simulink model "Citation"  (Simulink 10.0)
settings: Solver=ode5  StartTime=0.0  StopTime=700  FixedStep=0.01  RelTol=1e-3  EnableMultiTasking=on
values from neighbouring files (symbols this model uses):
  x0 = []    [cessnac550_3d_sfnc.m]
undefined symbols (not defined in the file or in its folder): chord, cv1, cv2, cv3, cv4, deltagmax1, deltagmax2, deltagmax3, deltagmax4, Deng, ealphag, ealphas, g0, hDME, hGS, kt1, kt2, kt3, lh, massinit, matbuaf, matdaf, matdam, matdbbf, matdeaf, matdgaf, matdqaf, matduaf, matdwaw, matedhr, mateif, matelhr, matemhr, matemv1, matemv2, matemve, matetam, mateuaf, matfaaf, matfaxl, matff, matibaf, matibmh, matipaf, matipmh, matiraf, matiuaf, matiwaf, matlaf, matlam, matleaf, matleam, matlgaf, matlqaf, matluaf, matmaaf, matmaam, matmaf, matmam, matmbbf ... (+77)
undefined symbols (not defined in the file): matibb
libraries: simulink x8, vrlib x1
(part 1 of 5)
settings Model: Creator=laurensvaneykeren  LastModifiedBy=mauro  ExtModeTrigMode=oneshot  ExtModeArmWhenConnect=off
settings DataIOCC: SignalLoggingName=sigsOut
settings OptimizationCC: BooleanDataType=off  ExpressionDepthLimit=2147483647
settings DebuggingCC: SaveWithParameterizedLinksMsg=none  SignalResolutionControl=TryResolveAllWithWarning  MultiTaskDSMMsg=warning  MultiTaskCondExecSysMsg=none  FcnCallInpInsideContextMsg=warning  StateNameClashWarn=warning
settings HardwareCC: TargetUnknown=on
settings RTWCC: SystemTargetFile=grt_malloc.tlc  GenCodeOnly=on  TemplateMakefile=grt_malloc_default_tmf
settings GRTTargetCC: UseMalloc=on

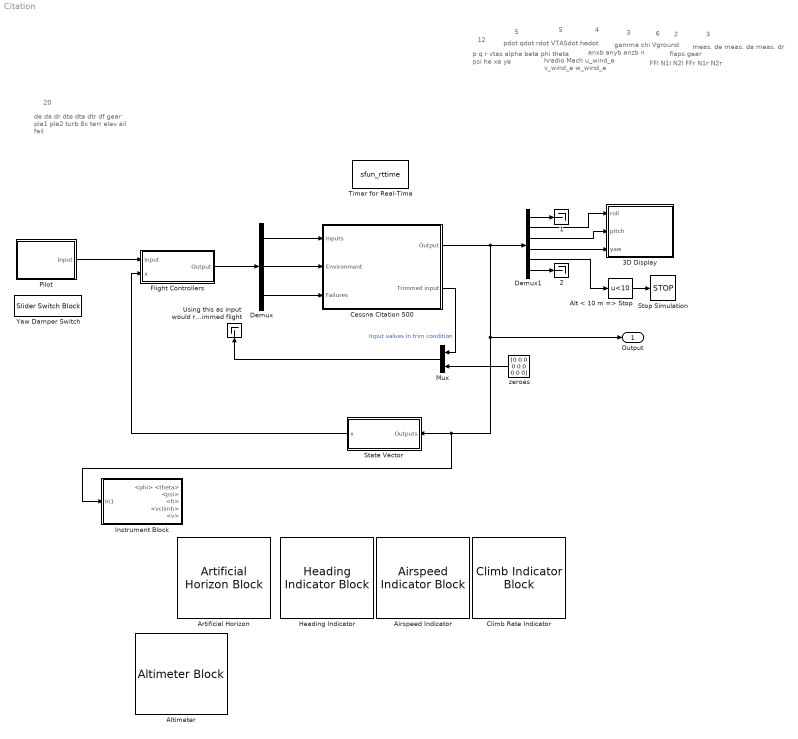
== system Citation ==
  note: de
      | da
      | dr
      | dte
      | dta
      | dtr
      | df
      | gear
      | pla1
      | pla2
      | turb 8x
      | terr elev
      | ail fail
  note: p
      | q
      | r
      | vtas
      | alpha
      | beta
      | phi
      | theta
      | psi
      | he
      | xe
      | ye
  note: pdot
      | qdot
      | rdot
      | VTASdot
      | hedot
  note: hradio
      | Mach
      | u_wind_e
      | v_wind_e
      | w_wind_e
  note: anxb
      | anyb
      | anzb
      | n
  note: gamma
      | chi
      | Vground
  note: flaps
      | gear
  note: FFl
      | N1l
      | N2l
      | FFr
      | N1r
      | N2r
  note: 12
  note: 5
  note: 5
  note: 4
  note: 3
  note: 6
  note: 2
  note: 20
  note: meas. de
      | meas. da
      | meas. dr
  note: 3
  1 : Terminator
  2 : Terminator
  3D Display : Subsystem
  Airspeed Indicator : AirspeedIndicatorBlock  ScaleMax=250  ScaleColors=DataTag1
  Alt < 10 m => Stop : Fcn  Expr=u<10
  Altimeter : AltimeterBlock
  Artificial Horizon : ArtificialHorizonBlock
  Cessna Citation 500 : Subsystem  mask(Citation Aircraft Model){trimdatafile=example.tri}
      mask prompts: trimdatafile "Trim Condition"
      mask init:
      | initcit;
      mask Display:
      | image(imread('Citation.jpg'))
      | port_label('input', 1, 'Inputs')
      | port_label('input', 2, 'Environment')
      | port_label('output', 1, 'Outputs')
      | port_label('output', 2, 'Trim inputs')
  Climb Rate Indicator : ClimbIndicatorBlock  ScaleMax=100
  Demux : Demux  Outputs=[10 9 1]
  Demux1 : Demux  Outputs=[6 1 1 1 1 30]
  Flight Controllers : Subsystem
  Heading Indicator : HeadingIndicatorBlock
  Instrument Block : Subsystem
  Mux : Mux  Inputs=2
  Pilot : Subsystem
  State Vector : Subsystem
  Stop Simulation : Stop
  Timer for Real-Time : S-Function  FunctionName=sfun_rttime  Parameters=1  SFunctionDeploymentMode=off  EnableBusSupport=off
  Using this as input would result in  trimmed flight : Terminator
  Yaw Damper Switch : SliderSwitchBlock  Values=DataTag7
  zeroes : Constant  Value=[0 0 0 0 0 0 0 0 0]
  Output : Outport
  wires:
  zeroes/1 -> Mux/2
  Mux/1 -> Using this as input would result in  trimmed flight/1
  Demux1/1 -> 1/1
  Demux1/2 -> 3D Display/1(roll)
  Demux1/3 -> 3D Display/2(pitch)
  Demux1/4 -> 3D Display/3(yaw)
  Alt < 10 m => Stop/1 -> Stop Simulation/1
  Demux1/6 -> 2/1
  Demux/1 -> Cessna Citation 500/1(Inputs)
  Demux/2 -> Cessna Citation 500/2(Environment)
  Cessna Citation 500/2(Trimmed input) -> Mux/1  "Input values in trim condition"
  Cessna Citation 500/1(Output) -> Demux1/1, Instrument Block/1(In1), State Vector/1(Outputs), Output/1
  Demux/3 -> Cessna Citation 500/3(Failures)
  State Vector/1(x) -> Flight Controllers/2(x)
  Pilot/1(Input) -> Flight Controllers/1(Input)
  Flight Controllers/1(Output) -> Demux/1
  Demux1/5 -> Alt < 10 m => Stop/1

== system Citation/3D Display ==
  roll : Inport
  pitch : Inport  Port=2
  yaw : Inport  Port=3
  Mux1 : Mux
  Position : Subsystem
  S-Function : S-Function  FunctionName=cessnac550_3d_sfnc  SFunctionDeploymentMode=off  EnableBusSupport=off
  Terminator : Terminator
  wires:
  roll/1 -> Mux1/1
  Position/1(Out1) -> Mux1/4
  pitch/1 -> Mux1/2
  yaw/1 -> Mux1/3
  Mux1/1 -> S-Function/1
  S-Function/1 -> Terminator/1

== system Citation/Cessna Citation 500 ==
  note: p
      | q
      | r
      | vtas
      | alpha
      | beta
      | phi
      | theta
      | psi
      | he
      | xe
      | ye
  note: de
      | da
      | dr
      | dte
      | dta
      | dtr
      | df
      | gear
      | pla1
      | pla2
  note: pdot
      | qdot
      | rdot
      | VTASdot
      | hedot
  note: hradio
      | Mach
      | u_wind_e
      | v_wind_e
      | w_wind_e
  note: anxb
      | anyb
      | anzb
      | n
  note: gamma
      | chi
      | Vground
  note: turb 8x
      | terr_elev
  note: flaps
      | gear
  note: de
      | da
      | dr
      | dte
      | dta
      | dtr
      | df
      | gear
      | pla1
      | pla2
  note: FFl
      | N1l
      | N2l
      | FFr
      | N1r
      | N2r
  note: ail fail
  note: meas. de
      | meas. da
      | meas. dr
  Inputs : Inport
  Environment : Inport  Port=2
  Failures : Inport  Port=3
  Actuators : Subsystem
  Citation model DASMAT : Subsystem
  Controllers : Subsystem
  Demux4 : Demux  Outputs=[8 2]
  Mux1 : Mux  Inputs=8
  Mux2 : Mux  Inputs=2
  Selector : Selector  InputPortWidth=12  IndexOptions=Index vector (dialog)  Indices=[10 11 12]  OutputSizes=1
  To File1 : ToFile  Filename=datapross\\data\\defl.mat  MatrixName=defl
  To File2 : ToFile  Filename=datapross\\data\\position.mat  MatrixName=pos
  trim conditions : Subsystem
  ua sel : Selector  IndexOptions=Index vector (dialog)  Indices=[5 6]  OutputSizes=1
  xdot sel : Selector  IndexOptions=Index vector (dialog)  Indices=[1 2 3 4 10]  OutputSizes=1
  yacc sel : Selector  IndexOptions=Index vector (dialog)  Indices=[4 5 6 15]  OutputSizes=1
  yair sel : Selector  IndexOptions=Index vector (dialog)  Indices=[6 9 22 23 24]  OutputSizes=1
  yfp sel : Selector  IndexOptions=Index vector (dialog)  Indices=[1 2 15]  OutputSizes=1
  ypp sel : Selector  IndexOptions=Index vector (dialog)  Indices=[2 3 4 13 14 15]  OutputSizes=1
  Output : Outport
  Trimmed input : Outport  Port=2
  wires:
  Mux1/1 -> Output/1
  Demux4/1 -> Citation model DASMAT/1(ua), ua sel/1
  Demux4/2 -> Citation model DASMAT/2(ut)
  Environment/1 -> Citation model DASMAT/3(Environment)
  Citation model DASMAT/3(yair) -> yair sel/1
  yair sel/1 -> Mux1/3
  Citation model DASMAT/2(xdot) -> xdot sel/1
  yacc sel/1 -> Mux1/4
  Citation model DASMAT/4(yacc) -> yacc sel/1
  yfp sel/1 -> Mux1/5
  Citation model DASMAT/5(yfp) -> yfp sel/1
  Actuators/1(Outputs) -> To File1/1, Demux4/1
  trim conditions/1(ua) -> Mux2/1
  trim conditions/2(ut) -> Mux2/2
  Mux2/1 -> Trimmed input/1
  Controllers/1(control inputs) -> Actuators/1(Inputs)
  ua sel/1 -> Mux1/7
  Citation model DASMAT/6(ypp) -> ypp sel/1
  ypp sel/1 -> Mux1/6
  Inputs/1 -> Controllers/2(inputs)
  Failures/1 -> Actuators/2(Failures)
  Actuators/2(Meas. Defl) -> Mux1/8
  xdot sel/1 -> Mux1/2
  Citation model DASMAT/1(x) -> Selector/1, Mux1/1, Controllers/1(state)
  Selector/1 -> To File2/1

== system Citation/Flight Controllers ==
  Input : Inport
  x : Inport  Port=2
  ANDI : Subsystem
  Classical : Subsystem
  Controller Switch : Subsystem
  INDI : Subsystem
  Multiport Switch : MultiPortSwitch  DataPortForDefault=Additional data port  DiagnosticForDefault=Warning
  To File : ToFile  Filename=datapross\\data\\output.mat  MatrixName=output
  To File1 : ToFile  Filename=datapross\\data\\input.mat  MatrixName=input
  Output : Outport
  wires:
  ANDI/1(Output) -> Multiport Switch/2
  x/1 -> INDI/2(x), Classical/2(x), ANDI/2(x)
  Controller Switch/1(Output) -> Multiport Switch/1
  Input/1 -> To File1/1, ANDI/1(Input), Classical/1(Input), INDI/1(Input), Multiport Switch/5
  INDI/1(Output) -> Multiport Switch/3
  Classical/1(Output) -> Multiport Switch/4
  Multiport Switch/1 -> To File/1, Output/1

== system Citation/Instrument Block ==
  In1 : Inport
  Demux : Demux  Outputs=[3 1 2 1 1 1 1 16 1 13]
  Demux5 : Demux  Outputs=2
  Gain : Gain  Gain=180/pi
  Gain2 : Gain  Gain=180/pi
  MATLAB Function : MATLAB Function  TreatAsAtomicUnit=on
  Mux3 : Mux  Inputs=2
  Mux4 : Mux  Inputs=2
  Product : Product
  Trigonometric Function : Trigonometry
  <phi> <theta> : Outport  VectorParamsAs1DForOutWhenUnconnected=off
  <psi> : Outport  Port=2  VectorParamsAs1DForOutWhenUnconnected=off
  <h> : Outport  Port=3  VectorParamsAs1DForOutWhenUnconnected=off
  <vclimb> : Outport  Port=4  VectorParamsAs1DForOutWhenUnconnected=off
  <v> : Outport  Port=5  VectorParamsAs1DForOutWhenUnconnected=off
  wires:
  Product/1 -> <vclimb>/1
  Mux3/1 -> Gain/1
  Trigonometric Function/1 -> Product/2
  Gain/1 -> Demux5/1
  Demux5/2 -> MATLAB Function/2(theta)
  MATLAB Function/2(theta_r) -> Mux4/2
  Demux5/1 -> MATLAB Function/1(phi)
  MATLAB Function/1(phi_r) -> Mux4/1
  Gain2/1 -> <psi>/1
  In1/1 -> Demux/1
  Mux4/1 -> <phi> <theta>/1
  Demux/2 -> <v>/1, Product/1
  Demux/4 -> Mux3/1
  Demux/5 -> Mux3/2
  Demux/6 -> Gain2/1
  Demux/7 -> <h>/1
  Demux/9 -> Trigonometric Function/1

== system Citation/Pilot ==
  note: de
      | da
      | dr
      | dte
      | dta
      | dtr
      | df
      | gear
      | pla1
      | pla2
      | turb 8x
      | terr elev
      | ail fail
  Joystick : Subsystem
  Mux : Mux  Inputs=13
  da trim : Constant  Value=0
  de trim : Constant  Value=0
  delta flaps : Constant  Value=0
  dr trim : Constant  Value=0
  gear (ON=1/OFF=0) : Constant  Value=0
  terr elev : Constant  Value=0
  turb 8x : Constant  Value=zeros(1,8)
  Input : Outport
  wires:
  Mux/1 -> Input/1
  Joystick/1(delta elevator) -> Mux/1
  Joystick/3(delta rudder) -> Mux/3
  da trim/1 -> Mux/5
  de trim/1 -> Mux/4
  Joystick/2(delta aileron) -> Mux/2
  turb 8x/1 -> Mux/11
  terr elev/1 -> Mux/12
  Joystick/4(Throttle setting) -> Mux/10, Mux/9
  gear (ON=1/OFF=0)/1 -> Mux/8
  dr trim/1 -> Mux/6
  delta flaps/1 -> Mux/7
  Joystick/5(Aileron failure) -> Mux/13

== system Citation/State Vector ==
  note: p
      | q
      | r
      | pdot
      | qdot
      | rdot
      | vtas
      | alpha
      | beta
      | u
      | v
      | w
      | phi
      | theta
      | rho
      | axb
      | ayb
      | azb
      | meas. de
      | meas. da
      | meas. dr
  note: 21
  note: p
      | q
      | r
  note: vtas
      | alpha
      | beta
  note: phi
      | theta
  note: he
  note: anxb
      | anyb
      | anzb
  note: meas. de
      | meas. da
      | meas. dr
  note: p
      | q
      | r
  note: vtas
      | alpha
      | beta
  note: phi
      | theta
  note: pdot
      | qdot
      | rdot
  note: u
      | v
      | w
  note: rho
  note: axb
      | ayb
      | azb
  note: meas. de
      | meas. da
      | meas. dr
  note: 6
  note: pdot
      | qdot
      | rdot
      | VTASdot
      | hedot
  note: 12
  note: meas. de
      | meas. da
      | meas. dr
  note: anxb
      | anyb
      | anzb
      | n
  note: FFl
      | N1l
      | N2l
      | FFr
      | N1r
      | N2r
  note: 5
  note: 3
  note: hradio
      | Mach
      | u_wind_e
      | v_wind_e
      | w_wind_e
  note: 3
  note: flaps
      | gear
  note: p
      | q
      | r
      | vtas
      | alpha
      | beta
      | phi
      | theta
      | psi
      | he
      | xe
      | ye
  note: 5
  note: gamma
      | chi
      | Vground
  note: 2
  note: 4
  Outputs : Inport
  Demux : Demux  Outputs=[3 3 2 1 1 12 3 12 3]
  Demux1 : Demux  Outputs=3
  Derivative : Derivative
  Gain : Gain  Gain=9.807
  MATLAB Function1 : MATLAB Function  TreatAsAtomicUnit=on
  MATLAB Function2 : MATLAB Function  TreatAsAtomicUnit=on
  Mux : Mux  Inputs=8
  Mux1 : Mux  Inputs=3
  Terminator1 : Terminator
  Terminator2 : Terminator
  Terminator3 : Terminator
  x : Outport
  wires:
  Demux/4 -> Terminator1/1
  Outputs/1 -> Demux/1
  Derivative/1 -> Mux/2
  Demux/6 -> Terminator2/1
  Demux/1 -> Mux/1, Derivative/1
  Demux/2 -> Demux1/1, Mux/3
  Demux1/1 -> MATLAB Function1/1(V)
  Demux1/2 -> MATLAB Function1/2(alpha)
  Demux1/3 -> MATLAB Function1/3(beta)
  MATLAB Function1/1(u) -> Mux1/1
  MATLAB Function1/2(v) -> Mux1/2
  MATLAB Function1/3(w) -> Mux1/3
  Mux1/1 -> Mux/4
  Demux/3 -> Mux/5
  MATLAB Function2/1(rho) -> Mux/6
  Demux/5 -> MATLAB Function2/1(h)
  Demux/7 -> Gain/1
  Gain/1 -> Mux/7
  Demux/8 -> Terminator3/1
  Demux/9 -> Mux/8
  Mux/1 -> x/1

== system Citation/3D Display/Position ==
  Mux2 : Mux  Inputs=3
  x : Constant  Value=0
  y : Constant  Value=0
  z : Constant  Value=0
  Out1 : Outport
  wires:
  y/1 -> Mux2/2
  z/1 -> Mux2/3
  x/1 -> Mux2/1
  Mux2/1 -> Out1/1

== system Citation/Cessna Citation 500/Actuators ==
  note: de
      | da
      | dr
      | dte
      | dta
      | dtr
      | df
      | gear
      | pla1
      | pla2
  note: de
      | da
      | dr
      | dte
      | dta
      | dtr
      | df
      | gear
      | pla1
      | pla2
  note: ail fail
  note: meas. de
      | meas. da
      | meas. dr
  Inputs : Inport
  Failures : Inport  Port=2
  Aileron Failure Dynamics : Subsystem
  Demux : Demux  Outputs=10
  Mux : Mux  Inputs=10
  Mux1 : Mux  Inputs=3
  Switch : Switch  Criteria=u2 > Threshold
  da : Subsystem
  da limits : Saturate  UpperLimit=0.65  LowerLimit=-0.65
  de : Subsystem
  de limits : Saturate  UpperLimit=0.26  LowerLimit=-0.35
  dr : Subsystem
  dr limits : Saturate  UpperLimit=0.38  LowerLimit=-0.38
  flaps : Subsystem
  gear : Subsystem
  Outputs : Outport
  Meas. Defl : Outport  Port=2
  wires:
  Inputs/1 -> Demux/1
  Mux/1 -> Outputs/1
  Demux/1 -> de/1(In)
  de/1(Out) -> de limits/1
  da/1(Out) -> da limits/1
  dr/1(Out) -> dr limits/1
  dr limits/1 -> Mux/3, Mux1/3
  de limits/1 -> Mux1/1, Mux/1
  Demux/8 -> gear/1(In)
  Demux/7 -> flaps/1(In)
  Demux/9 -> Mux/9
  Demux/10 -> Mux/10
  flaps/1(Out) -> Mux/7
  gear/1(Out) -> Mux/8
  Demux/4 -> Mux/4
  Demux/5 -> Mux/5
  Demux/6 -> Mux/6
  Failures/1 -> Switch/2
  Demux/3 -> dr/1(In)
  Switch/1 -> Mux/2
  Aileron Failure Dynamics/1(Out) -> Switch/1
  Demux/2 -> da/1(In)
  da limits/1 -> Mux1/2, Switch/3, Aileron Failure Dynamics/1(In)
  Mux1/1 -> Meas. Defl/1

== system Citation/Cessna Citation 500/Citation model DASMAT ==
  ua : Inport
  ut : Inport  Port=2
  Environment : Inport  Port=3
  AIRCRAFT MODEL : Subsystem
  Mux1 : Mux  Inputs=[8 2 8 12 8]
  Terminator_{16..19} (4 alike) : Terminator
  massinit : Constant  Value=massinit
  x : Outport
  xdot : Outport  Port=2
  yair : Outport  Port=3
  yacc : Outport  Port=4
  yfp : Outport  Port=5
  ypp : Outport  Port=6
  wires:
  AIRCRAFT MODEL/13(FMt) -> Terminator_19/1
  Mux1/1 -> yair/1
  AIRCRAFT MODEL/12(FMag) -> Terminator_17/1
  AIRCRAFT MODEL/11(FMa) -> Terminator_18/1
  AIRCRAFT MODEL/7(gust) -> Mux1/5
  AIRCRAFT MODEL/6(wind) -> Mux1/4
  AIRCRAFT MODEL/5(yad2) -> Mux1/3
  AIRCRAFT MODEL/4(yad1) -> Mux1/2
  AIRCRAFT MODEL/3(yatm) -> Mux1/1
  AIRCRAFT MODEL/2(xdot) -> xdot/1
  AIRCRAFT MODEL/1(x) -> x/1
  AIRCRAFT MODEL/10(ys) -> Terminator_16/1
  AIRCRAFT MODEL/9(yfp) -> yfp/1
  AIRCRAFT MODEL/8(yacc) -> yacc/1
  massinit/1 -> AIRCRAFT MODEL/3(massinit)
  ut/1 -> AIRCRAFT MODEL/2(ut)
  ua/1 -> AIRCRAFT MODEL/1(ua)
  Environment/1 -> AIRCRAFT MODEL/4(Environment)
  AIRCRAFT MODEL/14(ypp) -> ypp/1

== system Citation/Cessna Citation 500/Controllers ==
  state : Inport
  inputs : Inport  Port=2
  A/T disabled : Gain  Gain=0  SaturateOnIntegerOverflow=on  OutDataTypeStr=Inherit: Same as input  ParamDataTypeStr=Inherit: Same as input
  Yaw damper : Subsystem
  add controller outputs to pilot inputs : Sum  Inputs=|+|+|+|  SaturateOnIntegerOverflow=on
  auto throttle : Subsystem
  control inputs : Outport
  wires:
  state/1 -> Yaw damper/1(state), auto throttle/1(state)
  inputs/1 -> Yaw damper/2(inputs), add controller outputs to pilot inputs/3, auto throttle/2(inputs)
  add controller outputs to pilot inputs/1 -> control inputs/1
  Yaw damper/1(controller output) -> add controller outputs to pilot inputs/1
  auto throttle/1(controller output) -> A/T disabled/1
  A/T disabled/1 -> add controller outputs to pilot inputs/2

== system Citation/Cessna Citation 500/trim conditions ==
  PLA1/Tx1 : Constant  Value=ut0(1)
  PLA2/Tx2 : Constant  Value=ut0(2)
  control inputs : Mux  Inputs=8
      settings: DisplayOption=signals
  deltaa : Constant  Value=u0(2)
  deltae : Constant  Value=u0(1)
  deltaf : Constant  Value=u0(7)
  deltar : Constant  Value=u0(3)
  deltata : Constant  Value=u0(5)
  deltate : Constant  Value=u0(4)
  deltatr : Constant  Value=u0(6)
  engine inputs : Mux  Inputs=2
      settings: DisplayOption=signals
  lgsw : Constant  Value=u0(8)
  ua : Outport
  ut : Outport  Port=2
  wires:
  deltaf/1 -> control inputs/7  "df"
  engine inputs/1 -> ut/1
  deltatr/1 -> control inputs/6  "dtr"
  deltata/1 -> control inputs/5  "dta"
  control inputs/1 -> ua/1
  PLA1/Tx1/1 -> engine inputs/1  "pla1"
  PLA2/Tx2/1 -> engine inputs/2  "pla2"
  deltae/1 -> control inputs/1  "de"
  deltaa/1 -> control inputs/2  "da"
  deltar/1 -> control inputs/3  "dr"
  deltate/1 -> control inputs/4  "dte"
  lgsw/1 -> control inputs/8  "lg"

== system Citation/Flight Controllers/ANDI ==
  Input : Inport
  x : Inport  Port=2
  ANDI : Subsystem
  Demux : Demux  Outputs=[1 1 1 17]
  Memory : Memory  InitialCondition=[0, 0, 0, 0, 0, 0, 90.0, 0.0560, 0, 89.8590, 0, 5.0352, 0, 0.0037, 1.0065, 0.036, 0, -9.8008, -0.0248, 0, 0]
  Mux2 : Mux  Inputs=2
  Selector1 : Selector  InputPortWidth=3  IndexOptions=Index vector (dialog)  Indices=[2 1 3]  OutputSizes=1
  Output : Outport
  wires:
  Input/1 -> Demux/1
  Selector1/1 -> Mux2/1
  Demux/2 -> ANDI/2(p_ref)
  Demux/4 -> Mux2/2
  Demux/3 -> ANDI/4(beta_ref)
  Demux/1 -> ANDI/3(q_ref)
  Mux2/1 -> Output/1
  Memory/1 -> ANDI/1(x)
  x/1 -> Memory/1
  ANDI/1(Output) -> Selector1/1

== system Citation/Flight Controllers/Classical ==
  Input : Inport
  x : Inport  Port=2
  Classical : Subsystem
  Demux : Demux  Outputs=[1 1 1 17]
  Memory : Memory  InitialCondition=[0, 0, 0, 0, 0, 0, 90.0, 0.0560, 0, 89.8590, 0, 5.0352, 0, 0.0037, 1.0065, 0.036, 0, -9.8008, -0.0248, 0, 0]
  Mux2 : Mux  Inputs=2
  Selector1 : Selector  InputPortWidth=3  IndexOptions=Index vector (dialog)  Indices=[2 1 3]  OutputSizes=1
  Output : Outport
  wires:
  Input/1 -> Demux/1
  Selector1/1 -> Mux2/1
  Demux/2 -> Classical/2(p_ref)
  Demux/4 -> Mux2/2
  Demux/3 -> Classical/4(beta_ref)
  Demux/1 -> Classical/3(q_ref)
  Mux2/1 -> Output/1
  Memory/1 -> Classical/1(x)
  x/1 -> Memory/1
  Classical/1(Output) -> Selector1/1

== system Citation/Flight Controllers/Controller Switch ==
  Gain : Gain  Gain=[1;2;3;4]
  MATLAB Function : MATLAB Function  TreatAsAtomicUnit=on
  Memory : Memory  InitialCondition=1
  Output : Outport
  wires:
  [CSwitch] -> Gain/1
  Gain/1 -> MATLAB Function/1(input)
  MATLAB Function/1(output) -> Memory/1, Output/1
  Memory/1 -> MATLAB Function/2(prev)

== system Citation/Flight Controllers/INDI ==
  Input : Inport
  x : Inport  Port=2
  Demux : Demux  Outputs=[1 1 1 17]
  INDI : Subsystem
  Memory : Memory  InitialCondition=[0, 0, 0, 0, 0, 0, 90.0, 0.0560, 0, 89.8590, 0, 5.0352, 0, 0.0037, 1.0065, 0.036, 0, -9.8008, -0.0248, 0, 0]
  Mux2 : Mux  Inputs=2
  Selector1 : Selector  InputPortWidth=3  IndexOptions=Index vector (dialog)  Indices=[2 1 3]  OutputSizes=1
  Output : Outport
  wires:
  Input/1 -> Demux/1
  Selector1/1 -> Mux2/1
  Demux/2 -> INDI/2(p_ref)
  Demux/4 -> Mux2/2
  Demux/1 -> INDI/3(q_ref)
  Mux2/1 -> Output/1
  Memory/1 -> INDI/1(x)
  x/1 -> Memory/1
  INDI/1(Output) -> Selector1/1
  Demux/3 -> INDI/4(beta_ref)

== system Citation/Pilot/Joystick ==
  note: Button 3
  note: Button 2
  note: raw inputs
      | aileron [-0.6328,0.014,0.72] right+
      | elevator [-0.6973,-0.033,0.5725] backwards+
      | throttle [-0.6407,0,0.5317]bacwards+
      | rudder [-0.56,0.127,0.73] right+
  note: normalize inputs
      | aileron [-1,0,1] left+
      | elevator [-1,0,1] forward+
      | rudder [-1,0,1] left+
      | throttle [-1,0,1] forward+
  note: apply real limits
      | [deg]
      | [%]
  note: Convert to radians
      | [rad]
      | [%]
  Constant : Constant  Value=0
  Constant1 : Constant  Value=0
  Constant2 : Constant
  Constant3 : Constant  Value=0
  Dead Zone : DeadZone  LowerValue=-0.02  UpperValue=0.02  SaturateOnIntegerOverflow=on
  Dead Zone1 : DeadZone  LowerValue=-0.02  UpperValue=0.02  SaturateOnIntegerOverflow=on
  Dead Zone2 : DeadZone  LowerValue=-0.01  UpperValue=0.01  SaturateOnIntegerOverflow=on
  Demux : Demux  Outputs=2
  Demux1 : Demux
  Gain : Gain  Gain=-1  SaturateOnIntegerOverflow=on  OutDataTypeStr=Inherit: Same as input  ParamDataTypeStr=Inherit: Same as input
  Gain1 : Gain  Gain=-1  SaturateOnIntegerOverflow=on  OutDataTypeStr=Inherit: Same as input  ParamDataTypeStr=Inherit: Same as input
  Gain11 : Gain  Gain=pi/180  SaturateOnIntegerOverflow=on  OutDataTypeStr=Inherit: Same as input  ParamDataTypeStr=Inherit: Same as input
  Gain2 : Gain  Gain=-0.5  SaturateOnIntegerOverflow=on  OutDataTypeStr=Inherit: Same as input  ParamDataTypeStr=Inherit: Same as input
  Gain3 : Gain  Gain=-1  SaturateOnIntegerOverflow=on  OutDataTypeStr=Inherit: Same as input  ParamDataTypeStr=Inherit: Same as input
  Gain4 : Gain  Gain=37.24  SaturateOnIntegerOverflow=on  OutDataTypeStr=Inherit: Same as input  ParamDataTypeStr=Inherit: Same as input
  Gain5 : Gain  Gain=20  SaturateOnIntegerOverflow=on  OutDataTypeStr=Inherit: Same as input  ParamDataTypeStr=Inherit: Same as input
  Gain6 : Gain  SaturateOnIntegerOverflow=on  OutDataTypeStr=Inherit: Same as input  ParamDataTypeStr=Inherit: Same as input
  Gain7 : Gain  Gain=22  SaturateOnIntegerOverflow=on  OutDataTypeStr=Inherit: Same as input  ParamDataTypeStr=Inherit: Same as input
  Gain8 : Gain  Gain=pi/180  SaturateOnIntegerOverflow=on  OutDataTypeStr=Inherit: Same as input  ParamDataTypeStr=Inherit: Same as input
  Gain9 : Gain  Gain=pi/180  SaturateOnIntegerOverflow=on  OutDataTypeStr=Inherit: Same as input  ParamDataTypeStr=Inherit: Same as input
  Joystick Input : vrlib/Joystick Input  joyid=1  adjustports=on  forcefeed=off
      settings: SourceProductName=Simulink
  Selector : Selector  InputPortWidth=12  IndexOptions=Index vector (dialog)  Indices=[2 3]  OutputSizes=1
  Selector1 : Selector  InputPortWidth=12  IndexOptions=Index vector (dialog)  Indices=[7 9 11 12]  OutputSizes=1
  Sum{,1..3} (4 alike) : Sum  Inputs=-+|  SaturateOnIntegerOverflow=on
  Switch : Subsystem
  Terminator4 : Terminator
  delta elevator : Outport
  delta aileron : Outport  Port=2
  delta rudder : Outport  Port=3
  Throttle setting : Outport  Port=4
  Aileron failure : Outport  Port=5
  tag scope: CSwitch=global, FSwitch=global
  wires:
  Joystick Input/1 -> Demux1/1
  Joystick Input/2 -> Selector/1, Selector1/1
  Joystick Input/3 -> Terminator4/1
  Demux1/1 -> Sum/2
  Constant/1 -> Sum/1
  Constant1/1 -> Sum1/1
  Demux1/2 -> Sum1/2
  Constant2/1 -> Sum2/1
  Constant3/1 -> Sum3/1
  Sum/1 -> Dead Zone/1
  Gain/1 -> Gain4/1
  Sum1/1 -> Dead Zone1/1
  Gain1/1 -> Gain5/1
  Sum2/1 -> Gain2/1
  Sum3/1 -> Dead Zone2/1
  Gain3/1 -> Gain7/1
  Gain4/1 -> Gain8/1
  Gain5/1 -> Gain9/1
  Gain6/1 -> Throttle setting/1
  Gain7/1 -> Gain11/1
  Gain8/1 -> delta aileron/1
  Gain9/1 -> delta elevator/1
  Gain11/1 -> delta rudder/1
  Gain2/1 -> Gain6/1
  Demux1/4 -> Sum2/2
  Demux1/3 -> Sum3/2
  Dead Zone/1 -> Gain/1
  Dead Zone1/1 -> Gain1/1
  Dead Zone2/1 -> Gain3/1
  Demux/1 -> Switch/1(On)
  Demux/2 -> Switch/2(Off)
  Switch/1(Switch out) -> [FSwitch], Aileron failure/1
  Selector/1 -> Demux/1
  Selector1/1 -> [CSwitch]

== system Citation/Cessna Citation 500/Actuators/Aileron Failure Dynamics ==
  In : Inport
  Constant : Constant  Value=0.28
  Gain : Gain  Gain=0.5
  Sum : Sum  Inputs=|++
  Out : Outport
  wires:
  In/1 -> Gain/1
  Constant/1 -> Sum/2
  Gain/1 -> Sum/1
  Sum/1 -> Out/1

== system Citation/Cessna Citation 500/Actuators/da ==
  In : Inport
  Gain : Gain  Gain=13  SaturateOnIntegerOverflow=on  OutDataTypeStr=Inherit: Same as input  ParamDataTypeStr=Inherit: Same as input
  Integrator : Integrator  InitialCondition=u0(2)
  Sum : Sum  Inputs=|+-  SaturateOnIntegerOverflow=on
  Out : Outport
  wires:
  Integrator/1 -> Out/1, Sum/2
  In/1 -> Sum/1
  Sum/1 -> Gain/1
  Gain/1 -> Integrator/1

== system Citation/Cessna Citation 500/Actuators/de ==
  In : Inport
  Gain : Gain  Gain=13  SaturateOnIntegerOverflow=on  OutDataTypeStr=Inherit: Same as input  ParamDataTypeStr=Inherit: Same as input
  Integrator : Integrator  InitialCondition=u0(1)
  Sum : Sum  Inputs=|+-  SaturateOnIntegerOverflow=on
  Out : Outport
  wires:
  Integrator/1 -> Out/1, Sum/2
  In/1 -> Sum/1
  Sum/1 -> Gain/1
  Gain/1 -> Integrator/1

== system Citation/Cessna Citation 500/Actuators/dr ==
  In : Inport
  Gain : Gain  Gain=13  SaturateOnIntegerOverflow=on  OutDataTypeStr=Inherit: Same as input  ParamDataTypeStr=Inherit: Same as input
  Integrator : Integrator  InitialCondition=u0(3)
  Sum : Sum  Inputs=|+-  SaturateOnIntegerOverflow=on
  Out : Outport
  wires:
  Integrator/1 -> Out/1, Sum/2
  In/1 -> Sum/1
  Sum/1 -> Gain/1
  Gain/1 -> Integrator/1

== system Citation/Cessna Citation 500/Actuators/flaps ==
  In : Inport
  Gain : Gain  Gain=0.9  SaturateOnIntegerOverflow=on  OutDataTypeStr=Inherit: Same as input  ParamDataTypeStr=Inherit: Same as input
  Integrator : Integrator  InitialCondition=u0(7)
  Sum : Sum  Inputs=|+-  SaturateOnIntegerOverflow=on
  Out : Outport
  wires:
  Integrator/1 -> Out/1, Sum/2
  In/1 -> Sum/1
  Sum/1 -> Gain/1
  Gain/1 -> Integrator/1

== system Citation/Cessna Citation 500/Actuators/gear ==
  In : Inport
  Gain : Gain  Gain=0.6  SaturateOnIntegerOverflow=on  OutDataTypeStr=Inherit: Same as input  ParamDataTypeStr=Inherit: Same as input
  Integrator : Integrator  InitialCondition=u0(8)
  Sum : Sum  Inputs=|+-  SaturateOnIntegerOverflow=on
  Out : Outport
  wires:
  Integrator/1 -> Out/1, Sum/2
  In/1 -> Sum/1
  Sum/1 -> Gain/1
  Gain/1 -> Integrator/1

== system Citation/Cessna Citation 500/Citation model DASMAT/AIRCRAFT MODEL ==
  ua : Inport
  ut : Inport  Port=2
  massinit : Inport  Port=3
  Environment : Inport  Port=4
  AFM : Subsystem
  AIRDATA : Subsystem
  Demux : Demux  Outputs=[8 1]
  EFM : Subsystem
  EQM : Subsystem
  FM SORT : Subsystem
  GRAVITY : Subsystem
  LANDING GEAR : Subsystem
  OBSERVATIONS : Subsystem
  WIND/TURBULENCE : Subsystem
  x : Outport
  xdot : Outport  Port=2
  yatm : Outport  Port=3
  yad1 : Outport  Port=4
  yad2 : Outport  Port=5
  wind : Outport  Port=6
  gust : Outport  Port=7
  yacc : Outport  Port=8
  yfp : Outport  Port=9
  ys : Outport  Port=10
  FMa : Outport  Port=11
  FMag : Outport  Port=12
  FMt : Outport  Port=13
  ypp : Outport  Port=14
  wires:
  AFM/1(FMa) -> FM SORT/1(FMa), EQM/2(FMa)
  OBSERVATIONS/3(ys) -> ys/1
  OBSERVATIONS/2(yfp) -> yfp/1
  EQM/4(FMtot corrected) -> OBSERVATIONS/4(FMtot)
  EQM/3(yuvw) -> OBSERVATIONS/3(yuvw)
  EFM/1(FMt) -> FM SORT/3(FMt), FMt/1
  AFM/4(FMag) -> FM SORT/2(FMag), FMag/1
  ua/1 -> AFM/2(ua), LANDING GEAR/4(ua)
  ut/1 -> EFM/2(ut)
  OBSERVATIONS/1(yacc) -> yacc/1
  FM SORT/1(FMtot) -> EQM/1("FMtot ")
  EQM/5(FMa corrected) -> OBSERVATIONS/5(FMa), FMa/1
  AFM/2(FMadot) -> EQM/3(FMadot)
  AFM/3(FMbdot) -> EQM/4(FMbdot)
  GRAVITY/1(Fgr) -> FM SORT/4("Fgr "), OBSERVATIONS/6(Fgr)
  massinit/1 -> EFM/3(massinit), AFM/3(massinit), GRAVITY/2(massinit), EQM/5(massinit), OBSERVATIONS/7(massinit), LANDING GEAR/3(massinit)
  AIRDATA/3(yad2) -> EFM/6(yad2), AFM/5(yad2), yad2/1
  AIRDATA/2(yad1) -> AFM/4(yad1), EFM/5(yad1), yad1/1
  AIRDATA/1(yatm) -> yatm/1, GRAVITY/3(yatm), OBSERVATIONS/8(yatm), EFM/4(yatm), AFM/7(yatm)
  EQM/1(x) -> GRAVITY/1("x "), LANDING GEAR/1(x), EFM/1(x), AFM/1(x), WIND/TURBULENCE/1("x "), AIRDATA/1(x), x/1, OBSERVATIONS/1(x)
  WIND/TURBULENCE/1(wind) -> EQM/6(wind), wind/1
  EQM/2(xdot) -> xdot/1, OBSERVATIONS/2(xdot), LANDING GEAR/2(xdot)
  Environment/1 -> Demux/1
  Demux/1 -> gust/1, AFM/6(gust)
  Demux/2 -> AIRDATA/2(terrain  elevation), LANDING GEAR/5(terr elev)  "terrain elevation"
  LANDING GEAR/1(Fmt) -> FM SORT/5(Fgear)
  EFM/2(ypp) -> ypp/1

== system Citation/Cessna Citation 500/Controllers/Yaw damper ==
  state : Inport
  inputs : Inport  Port=2
  Gain : Gain  SaturateOnIntegerOverflow=on  OutDataTypeStr=Inherit: Same as input  ParamDataTypeStr=Inherit: Same as input
  Slider Switch : Constant  Value=0
  Switch : Switch  Criteria=u2 > Threshold
  Washout : TransferFcn  Numerator=[1 0]  Denominator=[1 1/4]
  Zeros : Constant  Value=[0 0 0 0 0 0 0 0 0 0]
  dr : Gain  Gain=[0 0 1 0 0 0 0 0 0 0]  SaturateOnIntegerOverflow=on  OutDataTypeStr=Inherit: Same as input  ParamDataTypeStr=Inherit: Same as input
  not used : Terminator
  r  sel : Selector  IndexOptions=Index vector (dialog)  Indices=[3]  OutputSizes=1
  controller output : Outport
  wires:
  Washout/1 -> Gain/1
  dr/1 -> Switch/1
  state/1 -> r  sel/1
  r  sel/1 -> Washout/1  "r"
  inputs/1 -> not used/1
  Gain/1 -> dr/1
  Switch/1 -> controller output/1
  Zeros/1 -> Switch/3
  Slider Switch/1 -> Switch/2

== system Citation/Cessna Citation 500/Controllers/auto throttle ==
  state : Inport
  inputs : Inport  Port=2
  Gain : Gain  Gain=0.5  SaturateOnIntegerOverflow=on  OutDataTypeStr=Inherit: Same as input  ParamDataTypeStr=Inherit: Same as input
  Saturation : Saturate  UpperLimit=1.0  LowerLimit=0.0
  Sum : Sum  Inputs=+-|  SaturateOnIntegerOverflow=on
  VTAS ref (trim value) : Constant  Value=x0(4)
  VTAS sel : Selector  IndexOptions=Index vector (dialog)  Indices=[4]  OutputSizes=1
  controller output is later added to pilot input! : Sum  Inputs=|+-  SaturateOnIntegerOverflow=on
  pla1&2 : Gain  Gain=[0 0 0 0 0 0 0 0 1 1]  SaturateOnIntegerOverflow=on  OutDataTypeStr=Inherit: Same as input  ParamDataTypeStr=Inherit: Same as input
  pla1&2 as well : Gain  Gain=[0 0 0 0 0 0 0 0 1 1]  SaturateOnIntegerOverflow=on  OutDataTypeStr=Inherit: Same as input  ParamDataTypeStr=Inherit: Same as input
  controller output : Outport
  wires:
  inputs/1 -> pla1&2 as well/1
  state/1 -> VTAS sel/1
  VTAS sel/1 -> Sum/2  "VTAS"
  VTAS ref (trim value)/1 -> Sum/1
  Sum/1 -> Gain/1
  pla1&2/1 -> controller output is later added to pilot input!/1
  Gain/1 -> Saturation/1
  controller output is later added to pilot input!/1 -> controller output/1
  Saturation/1 -> pla1&2/1
  pla1&2 as well/1 -> controller output is later added to pilot input!/2

== system Citation/Flight Controllers/ANDI/ANDI ==
  x : Inport
  p_ref : Inport  Port=2
  q_ref : Inport  Port=3
  beta_ref : Inport  Port=4
  AMI w/Loss : Subsystem
  AMI w/Stat Method : Subsystem
  Derivative : Derivative
  Derivative1 : Derivative
  Dynamic Inversion A : MATLAB Function  TreatAsAtomicUnit=on
  Dynamic Inversion B : MATLAB Function  TreatAsAtomicUnit=on
  Gain6 : Gain  Gain=-1
  Gain7 : Gain  Gain=-1
  Kynematic Inversion A : MATLAB Function  TreatAsAtomicUnit=on
  Kynematic Inversion B : MATLAB Function  TreatAsAtomicUnit=on
  Manual Switch : ManualSwitch
  Mux : Mux  Inputs=3
  PI Reset : Subsystem
  PI Reset1 : Subsystem
  PID Controller1 : simulink/Continuous/PID Controller  Controller=PI  Form=Parallel  TimeDomain=Continuous-time  SampleTime=-1  IntegratorMethod=Forward Euler  FilterMethod=Forward Euler  ControllerParametersSource=internal  P=8  I=2  D=0  UseFilter=on  N=100  TunerSelectOption=Transfer Function Based (PID Tuner App)  InitialConditionSource=internal  InitialConditionForIntegrator=0  InitialConditionForFilter=0  DifferentiatorICPrevScaledInput=0  ExternalReset=rising  TrackingMode=off  Kt=1  LimitOutput=off  UpperSaturationLimit=inf  LowerSaturationLimit=-inf  LinearizeAsGain=on  AntiWindupMode=none  Kb=1  POutMin=[]  POutMax=[]  IOutMin=[]  IOutMax=[]  DOutMin=[]  DOutMax=[]  NOutMin=[]  NOutMax=[]  SumOutMin=[]  SumOutMax=[]  SaturationOutMin=[]  SaturationOutMax=[]  PParamMin=[]  PParamMax=[]  IParamMin=[]  IParamMax=[]  DParamMin=[]  DParamMax=[]  NParamMin=[]  NParamMax=[]  KbParamMin=[]  KbParamMax=[]  KtParamMin=[]  KtParamMax=[]  KbOutMin=[]  KbOutMax=[]  KtOutMin=[]  KtOutMax=[]  IntegratorOutMin=[]  IntegratorOutMax=[]  FilterOutMin=[]  FilterOutMax=[]  SumI1OutMin=[]  SumI1OutMax=[]  SumI2OutMin=[]  SumI2OutMax=[]  SumI3OutMin=[]  SumI3OutMax=[]  SumI4OutMin=[]  SumI4OutMax=[]  SumDOutMin=[]  SumDOutMax=[]  DifferentiatorOutMin=[]  DifferentiatorOutMax=[]  FilterDiffOutCoefMin=[]  FilterDiffOutCoefMax=[]  ReciprocalOutMin=[]  ReciprocalOutMax=[]  SumDenOutMin=[]  SumDenOutMax=[]  SumNumOutMin=[]  SumNumOutMax=[]  DivideOutMin=[]  DivideOutMax=[]  IntegratorContinuousStateAttributes=''  IntegratorStateMustResolveToSignalObject=off  IntegratorRTWStateStorageClass=Auto  FilterContinuousStateAttributes=''  FilterStateMustResolveToSignalObject=off  FilterRTWStateStorageClass=Auto  ParallelPVariant=InternalParameters  IdealPVariant=Disabled  IVariant=InternalParameters  DVariant=Disabled  IntegratorVariant=Continuous  SatVariant=Disabled  AWVariant=Passthrough  PCopyVariant=Disabled  TRVariant=Disabled  FdbkBlocksVariant=Forward  IdealPFdbkVariant=Disabled  SatFdbkVariant=Disabled  DerivativeFilterVariant=Disabled  NVariant=Disabled  NCopyVariant=Disabled_SignalSpec  FilterICVariant=Disabled  IntegratorICVariant=InternalICs  ExternalResetVariant=ExternalReset  TRSumVariant=Passthrough  SumFdbkVariant=Disabled  SumVariant=Sum_PI
  PID Controller2 : simulink/Continuous/PID Controller  Controller=PI  Form=Parallel  TimeDomain=Continuous-time  SampleTime=-1  IntegratorMethod=Forward Euler  FilterMethod=Forward Euler  ControllerParametersSource=internal  P=1  I=0.5  D=0  UseFilter=on  N=100  TunerSelectOption=Transfer Function Based (PID Tuner App)  InitialConditionSource=internal  InitialConditionForIntegrator=0  InitialConditionForFilter=0  DifferentiatorICPrevScaledInput=0  ExternalReset=rising  TrackingMode=off  Kt=1  LimitOutput=off  UpperSaturationLimit=inf  LowerSaturationLimit=-inf  LinearizeAsGain=on  AntiWindupMode=none  Kb=1  POutMin=[]  POutMax=[]  IOutMin=[]  IOutMax=[]  DOutMin=[]  DOutMax=[]  NOutMin=[]  NOutMax=[]  SumOutMin=[]  SumOutMax=[]  SaturationOutMin=[]  SaturationOutMax=[]  PParamMin=[]  PParamMax=[]  IParamMin=[]  IParamMax=[]  DParamMin=[]  DParamMax=[]  NParamMin=[]  NParamMax=[]  KbParamMin=[]  KbParamMax=[]  KtParamMin=[]  KtParamMax=[]  KbOutMin=[]  KbOutMax=[]  KtOutMin=[]  KtOutMax=[]  IntegratorOutMin=[]  IntegratorOutMax=[]  FilterOutMin=[]  FilterOutMax=[]  SumI1OutMin=[]  SumI1OutMax=[]  SumI2OutMin=[]  SumI2OutMax=[]  SumI3OutMin=[]  SumI3OutMax=[]  SumI4OutMin=[]  SumI4OutMax=[]  SumDOutMin=[]  SumDOutMax=[]  DifferentiatorOutMin=[]  DifferentiatorOutMax=[]  FilterDiffOutCoefMin=[]  FilterDiffOutCoefMax=[]  ReciprocalOutMin=[]  ReciprocalOutMax=[]  SumDenOutMin=[]  SumDenOutMax=[]  SumNumOutMin=[]  SumNumOutMax=[]  DivideOutMin=[]  DivideOutMax=[]  IntegratorContinuousStateAttributes=''  IntegratorStateMustResolveToSignalObject=off  IntegratorRTWStateStorageClass=Auto  FilterContinuousStateAttributes=''  FilterStateMustResolveToSignalObject=off  FilterRTWStateStorageClass=Auto  ParallelPVariant=InternalParameters  IdealPVariant=Disabled  IVariant=InternalParameters  DVariant=Disabled  IntegratorVariant=Continuous  SatVariant=Disabled  AWVariant=Passthrough  PCopyVariant=Disabled  TRVariant=Disabled  FdbkBlocksVariant=Forward  IdealPFdbkVariant=Disabled  SatFdbkVariant=Disabled  DerivativeFilterVariant=Disabled  NVariant=Disabled  NCopyVariant=Disabled_SignalSpec  FilterICVariant=Disabled  IntegratorICVariant=InternalICs  ExternalResetVariant=ExternalReset  TRSumVariant=Passthrough  SumFdbkVariant=Disabled  SumVariant=Sum_PI
  Selector : Selector  InputPortWidth=21  IndexOptions=Index vector (dialog)  Indices=[1 2 3]  OutputSizes=1
  Selector1 : Selector  InputPortWidth=21  IndexOptions=Index vector (dialog)  Indices=[9]  OutputSizes=1
  Sum{,1,3..4} (4 alike) : Sum  Inputs=|+-
  Sum5 : Sum  Inputs=++|
  Sum6 : Sum  Inputs=++|
  Transfer Fcn : TransferFcn  Numerator=[15]  Denominator=[1 15]
  Transfer Fcn1 : TransferFcn  Numerator=[10]  Denominator=[1 10]
  Transfer Fcn2 : TransferFcn  Numerator=[0.5]  Denominator=[1 0.5]
  Output : Outport
  wires:
  Dynamic Inversion A/1(a) -> Sum/2
  Derivative/1 -> Sum6/1
  Sum3/1 -> Kynematic Inversion B/1(Y)
  Sum/1 -> Dynamic Inversion B/1(Y)
  Manual Switch/1 -> Dynamic Inversion A/2(p_k), Dynamic Inversion B/3(p_k)
  AMI w/Stat Method/1(p_k) -> Manual Switch/1
  AMI w/Loss/1(p_k) -> Manual Switch/2
  Sum1/1 -> PID Controller1/1
  Selector/1 -> Sum1/2
  Kynematic Inversion A/1(a) -> Sum3/2
  Kynematic Inversion B/1(U) -> Sum1/1, Derivative/1
  Dynamic Inversion B/1(U) -> Output/1
  Sum6/1 -> Sum/1
  Gain6/1 -> Transfer Fcn/1
  Gain7/1 -> Transfer Fcn1/1
  beta_ref/1 -> Transfer Fcn2/1
  p_ref/1 -> Gain6/1
  Mux/1 -> Sum3/1
  q_ref/1 -> Gain7/1
  x/1 -> AMI w/Stat Method/1(x), AMI w/Loss/1(x), Dynamic Inversion B/2(x), Selector/1, Kynematic Inversion B/2(x), Selector1/1, Kynematic Inversion A/1(x), Dynamic Inversion A/1(x)
  Sum4/1 -> PID Controller2/1
  Derivative1/1 -> Sum5/1
  Sum5/1 -> Mux/3
  Transfer Fcn/1 -> Mux/1
  Selector1/1 -> Sum4/2
  Transfer Fcn2/1 -> Sum4/1, Derivative1/1
  Transfer Fcn1/1 -> Mux/2
  PID Controller2/1 -> Sum5/2
  PID Controller1/1 -> Sum6/2
  PI Reset/1(Out) -> PID Controller2/2
  PI Reset1/1(Out) -> PID Controller1/2

== system Citation/Flight Controllers/Classical/Classical ==
  x : Inport
  p_ref : Inport  Port=2
  q_ref : Inport  Port=3
  beta_ref : Inport  Port=4
  Demux : Demux  Outputs=3
  Gain6 : Gain  Gain=-1
  Gain7 : Gain  Gain=-1
  Mux : Mux  Inputs=3
  Mux2 : Mux  Inputs=3
  PI Reset : Subsystem
  PI Reset1 : Subsystem
  PID Controller : simulink/Continuous/PID Controller  Controller=PI  Form=Parallel  TimeDomain=Continuous-time  SampleTime=-1  IntegratorMethod=Forward Euler  FilterMethod=Forward Euler  ControllerParametersSource=internal  P=-1  I=-0.1  D=0  UseFilter=on  N=100  TunerSelectOption=Transfer Function Based (PID Tuner App)  InitialConditionSource=internal  InitialConditionForIntegrator=0  InitialConditionForFilter=0  DifferentiatorICPrevScaledInput=0  ExternalReset=rising  TrackingMode=off  Kt=1  LimitOutput=off  UpperSaturationLimit=inf  LowerSaturationLimit=-inf  LinearizeAsGain=on  AntiWindupMode=none  Kb=1  POutMin=[]  POutMax=[]  IOutMin=[]  IOutMax=[]  DOutMin=[]  DOutMax=[]  NOutMin=[]  NOutMax=[]  SumOutMin=[]  SumOutMax=[]  SaturationOutMin=[]  SaturationOutMax=[]  PParamMin=[]  PParamMax=[]  IParamMin=[]  IParamMax=[]  DParamMin=[]  DParamMax=[]  NParamMin=[]  NParamMax=[]  KbParamMin=[]  KbParamMax=[]  KtParamMin=[]  KtParamMax=[]  KbOutMin=[]  KbOutMax=[]  KtOutMin=[]  KtOutMax=[]  IntegratorOutMin=[]  IntegratorOutMax=[]  FilterOutMin=[]  FilterOutMax=[]  SumI1OutMin=[]  SumI1OutMax=[]  SumI2OutMin=[]  SumI2OutMax=[]  SumI3OutMin=[]  SumI3OutMax=[]  SumI4OutMin=[]  SumI4OutMax=[]  SumDOutMin=[]  SumDOutMax=[]  DifferentiatorOutMin=[]  DifferentiatorOutMax=[]  FilterDiffOutCoefMin=[]  FilterDiffOutCoefMax=[]  ReciprocalOutMin=[]  ReciprocalOutMax=[]  SumDenOutMin=[]  SumDenOutMax=[]  SumNumOutMin=[]  SumNumOutMax=[]  DivideOutMin=[]  DivideOutMax=[]  IntegratorContinuousStateAttributes=''  IntegratorStateMustResolveToSignalObject=off  IntegratorRTWStateStorageClass=Auto  FilterContinuousStateAttributes=''  FilterStateMustResolveToSignalObject=off  FilterRTWStateStorageClass=Auto  ParallelPVariant=InternalParameters  IdealPVariant=Disabled  IVariant=InternalParameters  DVariant=Disabled  IntegratorVariant=Continuous  SatVariant=Disabled  AWVariant=Passthrough  PCopyVariant=Disabled  TRVariant=Disabled  FdbkBlocksVariant=Forward  IdealPFdbkVariant=Disabled  SatFdbkVariant=Disabled  DerivativeFilterVariant=Disabled  NVariant=Disabled  NCopyVariant=Disabled_SignalSpec  FilterICVariant=Disabled  IntegratorICVariant=InternalICs  ExternalResetVariant=ExternalReset  TRSumVariant=Passthrough  SumFdbkVariant=Disabled  SumVariant=Sum_PI
  PID Controller1 : simulink/Continuous/PID Controller  Controller=PI  Form=Parallel  TimeDomain=Continuous-time  SampleTime=-1  IntegratorMethod=Forward Euler  FilterMethod=Forward Euler  ControllerParametersSource=internal  P=-2  I=-0.1  D=0  UseFilter=on  N=100  TunerSelectOption=Transfer Function Based (PID Tuner App)  InitialConditionSource=internal  InitialConditionForIntegrator=0  InitialConditionForFilter=0  DifferentiatorICPrevScaledInput=0  ExternalReset=rising  TrackingMode=off  Kt=1  LimitOutput=off  UpperSaturationLimit=inf  LowerSaturationLimit=-inf  LinearizeAsGain=on  AntiWindupMode=none  Kb=1  POutMin=[]  POutMax=[]  IOutMin=[]  IOutMax=[]  DOutMin=[]  DOutMax=[]  NOutMin=[]  NOutMax=[]  SumOutMin=[]  SumOutMax=[]  SaturationOutMin=[]  SaturationOutMax=[]  PParamMin=[]  PParamMax=[]  IParamMin=[]  IParamMax=[]  DParamMin=[]  DParamMax=[]  NParamMin=[]  NParamMax=[]  KbParamMin=[]  KbParamMax=[]  KtParamMin=[]  KtParamMax=[]  KbOutMin=[]  KbOutMax=[]  KtOutMin=[]  KtOutMax=[]  IntegratorOutMin=[]  IntegratorOutMax=[]  FilterOutMin=[]  FilterOutMax=[]  SumI1OutMin=[]  SumI1OutMax=[]  SumI2OutMin=[]  SumI2OutMax=[]  SumI3OutMin=[]  SumI3OutMax=[]  SumI4OutMin=[]  SumI4OutMax=[]  SumDOutMin=[]  SumDOutMax=[]  DifferentiatorOutMin=[]  DifferentiatorOutMax=[]  FilterDiffOutCoefMin=[]  FilterDiffOutCoefMax=[]  ReciprocalOutMin=[]  ReciprocalOutMax=[]  SumDenOutMin=[]  SumDenOutMax=[]  SumNumOutMin=[]  SumNumOutMax=[]  DivideOutMin=[]  DivideOutMax=[]  IntegratorContinuousStateAttributes=''  IntegratorStateMustResolveToSignalObject=off  IntegratorRTWStateStorageClass=Auto  FilterContinuousStateAttributes=''  FilterStateMustResolveToSignalObject=off  FilterRTWStateStorageClass=Auto  ParallelPVariant=InternalParameters  IdealPVariant=Disabled  IVariant=InternalParameters  DVariant=Disabled  IntegratorVariant=Continuous  SatVariant=Disabled  AWVariant=Passthrough  PCopyVariant=Disabled  TRVariant=Disabled  FdbkBlocksVariant=Forward  IdealPFdbkVariant=Disabled  SatFdbkVariant=Disabled  DerivativeFilterVariant=Disabled  NVariant=Disabled  NCopyVariant=Disabled_SignalSpec  FilterICVariant=Disabled  IntegratorICVariant=InternalICs  ExternalResetVariant=ExternalReset  TRSumVariant=Passthrough  SumFdbkVariant=Disabled  SumVariant=Sum_PI
  PID Controller2 : simulink/Continuous/PID Controller  Controller=PI  Form=Parallel  TimeDomain=Continuous-time  SampleTime=-1  IntegratorMethod=Forward Euler  FilterMethod=Forward Euler  ControllerParametersSource=internal  P=-2  I=-0.1  D=0  UseFilter=on  N=100  TunerSelectOption=Transfer Function Based (PID Tuner App)  InitialConditionSource=internal  InitialConditionForIntegrator=0  InitialConditionForFilter=0  DifferentiatorICPrevScaledInput=0  ExternalReset=rising  TrackingMode=off  Kt=1  LimitOutput=off  UpperSaturationLimit=inf  LowerSaturationLimit=-inf  LinearizeAsGain=on  AntiWindupMode=none  Kb=1  POutMin=[]  POutMax=[]  IOutMin=[]  IOutMax=[]  DOutMin=[]  DOutMax=[]  NOutMin=[]  NOutMax=[]  SumOutMin=[]  SumOutMax=[]  SaturationOutMin=[]  SaturationOutMax=[]  PParamMin=[]  PParamMax=[]  IParamMin=[]  IParamMax=[]  DParamMin=[]  DParamMax=[]  NParamMin=[]  NParamMax=[]  KbParamMin=[]  KbParamMax=[]  KtParamMin=[]  KtParamMax=[]  KbOutMin=[]  KbOutMax=[]  KtOutMin=[]  KtOutMax=[]  IntegratorOutMin=[]  IntegratorOutMax=[]  FilterOutMin=[]  FilterOutMax=[]  SumI1OutMin=[]  SumI1OutMax=[]  SumI2OutMin=[]  SumI2OutMax=[]  SumI3OutMin=[]  SumI3OutMax=[]  SumI4OutMin=[]  SumI4OutMax=[]  SumDOutMin=[]  SumDOutMax=[]  DifferentiatorOutMin=[]  DifferentiatorOutMax=[]  FilterDiffOutCoefMin=[]  FilterDiffOutCoefMax=[]  ReciprocalOutMin=[]  ReciprocalOutMax=[]  SumDenOutMin=[]  SumDenOutMax=[]  SumNumOutMin=[]  SumNumOutMax=[]  DivideOutMin=[]  DivideOutMax=[]  IntegratorContinuousStateAttributes=''  IntegratorStateMustResolveToSignalObject=off  IntegratorRTWStateStorageClass=Auto  FilterContinuousStateAttributes=''  FilterStateMustResolveToSignalObject=off  FilterRTWStateStorageClass=Auto  ParallelPVariant=InternalParameters  IdealPVariant=Disabled  IVariant=InternalParameters  DVariant=Disabled  IntegratorVariant=Continuous  SatVariant=Disabled  AWVariant=Passthrough  PCopyVariant=Disabled  TRVariant=Disabled  FdbkBlocksVariant=Forward  IdealPFdbkVariant=Disabled  SatFdbkVariant=Disabled  DerivativeFilterVariant=Disabled  NVariant=Disabled  NCopyVariant=Disabled_SignalSpec  FilterICVariant=Disabled  IntegratorICVariant=InternalICs  ExternalResetVariant=ExternalReset  TRSumVariant=Passthrough  SumFdbkVariant=Disabled  SumVariant=Sum_PI
  PID Controller3 : simulink/Continuous/PID Controller  Controller=PI  Form=Parallel  TimeDomain=Continuous-time  SampleTime=-1  IntegratorMethod=Forward Euler  FilterMethod=Forward Euler  ControllerParametersSource=internal  P=-1  I=-0.5  D=0  UseFilter=on  N=100  TunerSelectOption=Transfer Function Based (PID Tuner App)  InitialConditionSource=internal  InitialConditionForIntegrator=0  InitialConditionForFilter=0  DifferentiatorICPrevScaledInput=0  ExternalReset=rising  TrackingMode=off  Kt=1  LimitOutput=off  UpperSaturationLimit=inf  LowerSaturationLimit=-inf  LinearizeAsGain=on  AntiWindupMode=none  Kb=1  POutMin=[]  POutMax=[]  IOutMin=[]  IOutMax=[]  DOutMin=[]  DOutMax=[]  NOutMin=[]  NOutMax=[]  SumOutMin=[]  SumOutMax=[]  SaturationOutMin=[]  SaturationOutMax=[]  PParamMin=[]  PParamMax=[]  IParamMin=[]  IParamMax=[]  DParamMin=[]  DParamMax=[]  NParamMin=[]  NParamMax=[]  KbParamMin=[]  KbParamMax=[]  KtParamMin=[]  KtParamMax=[]  KbOutMin=[]  KbOutMax=[]  KtOutMin=[]  KtOutMax=[]  IntegratorOutMin=[]  IntegratorOutMax=[]  FilterOutMin=[]  FilterOutMax=[]  SumI1OutMin=[]  SumI1OutMax=[]  SumI2OutMin=[]  SumI2OutMax=[]  SumI3OutMin=[]  SumI3OutMax=[]  SumI4OutMin=[]  SumI4OutMax=[]  SumDOutMin=[]  SumDOutMax=[]  DifferentiatorOutMin=[]  DifferentiatorOutMax=[]  FilterDiffOutCoefMin=[]  FilterDiffOutCoefMax=[]  ReciprocalOutMin=[]  ReciprocalOutMax=[]  SumDenOutMin=[]  SumDenOutMax=[]  SumNumOutMin=[]  SumNumOutMax=[]  DivideOutMin=[]  DivideOutMax=[]  IntegratorContinuousStateAttributes=''  IntegratorStateMustResolveToSignalObject=off  IntegratorRTWStateStorageClass=Auto  FilterContinuousStateAttributes=''  FilterStateMustResolveToSignalObject=off  FilterRTWStateStorageClass=Auto  ParallelPVariant=InternalParameters  IdealPVariant=Disabled  IVariant=InternalParameters  DVariant=Disabled  IntegratorVariant=Continuous  SatVariant=Disabled  AWVariant=Passthrough  PCopyVariant=Disabled  TRVariant=Disabled  FdbkBlocksVariant=Forward  IdealPFdbkVariant=Disabled  SatFdbkVariant=Disabled  DerivativeFilterVariant=Disabled  NVariant=Disabled  NCopyVariant=Disabled_SignalSpec  FilterICVariant=Disabled  IntegratorICVariant=InternalICs  ExternalResetVariant=ExternalReset  TRSumVariant=Passthrough  SumFdbkVariant=Disabled  SumVariant=Sum_PI
  Selector : Selector  InputPortWidth=21  IndexOptions=Index vector (dialog)  Indices=[9]  OutputSizes=1
  Selector1 : Selector  InputPortWidth=21  IndexOptions=Index vector (dialog)  Indices=[1 2 3]  OutputSizes=1
  Sum1 : Sum  Inputs=|+-
  Sum2 : Sum  Inputs=|+-
  Output : Outport
  wires:
  p_ref/1 -> Gain6/1
  q_ref/1 -> Gain7/1
  beta_ref/1 -> Sum1/1
  Selector/1 -> Sum1/2
  x/1 -> Selector1/1, Selector/1
  Sum1/1 -> PID Controller/1
  Gain6/1 -> Mux/1
  Gain7/1 -> Mux/2
  PID Controller/1 -> Mux/3
  Mux/1 -> Sum2/1
  Selector1/1 -> Sum2/2
  Demux/1 -> PID Controller3/1
  Sum2/1 -> Demux/1
  PID Controller3/1 -> Mux2/1
  Demux/2 -> PID Controller2/1
  PID Controller2/1 -> Mux2/2
  Demux/3 -> PID Controller1/1
  PID Controller1/1 -> Mux2/3
  Mux2/1 -> Output/1
  PI Reset/1(Out) -> PID Controller/2
  PI Reset1/1(Out) -> PID Controller1/2, PID Controller2/2, PID Controller3/2
